simulink model "ModeloCodesys"  (R2020b)
settings: Solver=FixedStepAuto  StartTime=0.0  StopTime=inf  FixedStep=1e-2  MaxStep=1e-4  RelTol=1e-3
model workspace (MAT data in the model file):
  sensor_carga : Simulink.Parameter (value not decoded)
values from neighbouring files (symbols this model uses):
  bcx = 1000e3    (= 1000000)    [Datos_simulacion.m]
  bcy = 500e3    (= 500000)    [Datos_simulacion.m]
  beq_tc = (bv_c+beq_cel)/Rw^2    (= 27000)    [Datos_simulacion.m]
  beq_ti = (b_h+beq_iel)/Rd^2    (= 28800)    [Datos_simulacion.m]
  bw = 30e3    (= 30000)    [Datos_simulacion.m]
  g = 9.80665    [Datos_simulacion.m]
  i_c = 15    [Datos_simulacion.m]
  i_i = 30    [Datos_simulacion.m]
  Kcd = Meq_c*polo_c*n    (= 472500)    [Datos_simulacion.m]
  Kci = Kcp*polo_c/n    (= 1938936.66179)    [Datos_simulacion.m]
  Kcp = Kcd*polo_c    (= 1513396.48861)    [Datos_simulacion.m]
  Kcy = 1.3e9    (= 1300000000)    [Datos_simulacion.m]
  Kid = Kcp*polo_i/n    (= 1815537.84919)    [Datos_simulacion.m]
  Kii = Meq_i*polo_i*n    (= 360000)    [Datos_simulacion.m]
  Kip = Kcd*polo_i    (= 1417080.12441)    [Datos_simulacion.m]
  Kw = 1800e3    (= 1800000)    [Datos_simulacion.m]
  Meq_c = m_c+Jeq_c/Rw^2    (= 59008)    [Datos_simulacion.m]
  Meq_i = m_h+Jeq_i/Rd^2    (= 48014.2222222)    [Datos_simulacion.m]
  Rd = 0.75    [Datos_simulacion.m]
  Rw = 0.5    [Datos_simulacion.m]
  Tau = 1e-3    (= 0.001)    [Datos_simulacion.m]
libraries: simulink x2, fuzblock x1, pid_lib x1, dspswit3 x1
(part 2 of 2)

== matlab function ModeloCodesys/Algoritmos de busqueda de camino y interpolacion/Interpolador ==
  data: wayPoints input size=2,100; q output size=[2,1000000]; velMaxX input; velMaxY input
function q  = Interp(wayPoints,velMaxX,velMaxY)
coder.extrinsic('plot')
pendiente_ant=0;
cont_p=1;
wayPoints=wayPoints([2,1],:);
wayPoints=flip(wayPoints,2);
wayPoints(2,:)=(wayPoints(2,:)-65)*-1;
for i=1:length(wayPoints)-1
    pendiente=(wayPoints(2,i)-wayPoints(2,i+1))/(wayPoints(1,i)-wayPoints(1,i+1));
    if pendiente_ant~=pendiente
        cont_p=cont_p+1;
    end
    pendiente_ant=pendiente;
end
wayPoints1=zeros(2,cont_p);
cont_p2=0;
for i=1:length(wayPoints(1,:))-1
    pendiente=(wayPoints(2,i)-wayPoints(2,i+1))/(wayPoints(1,i)-wayPoints(1,i+1));
    if pendiente_ant~=pendiente
    cont_p2=cont_p2+1;
    wayPoints1(:,cont_p2)=wayPoints(:,i);
    end
    pendiente_ant=pendiente;
end
wayPoints1(:,end)=wayPoints(:,end);
wayPoints1(:,1)=wayPoints(:,1);
figure(10)
plot(wayPoints1(1,:),wayPoints1(2,:))   
vx_max=velMaxX;
vy_max=velMaxY;
timePoints1=zeros(1,length(wayPoints1));
tiempo_ant=0;
for i=1:length(wayPoints1(1,:))-1
    restaX=abs(wayPoints1(1,i+1)-wayPoints1(1,i));
    restaY=abs(wayPoints1(2,i+1)-wayPoints1(2,i));
    timex=restaX/(vx_max/2.5);
    timey=restaY/(vy_max/2.5);
    if timex>timey
    timePoints1(i+1)=restaX/(vx_max/4)+tiempo_ant;
    elseif timex<timey
    timePoints1(i+1)=restaY/(vy_max/4)+tiempo_ant;
    else
     timePoints1(i+1)=restaX/(vx_max/4)+tiempo_ant;    
    end
    tiempo_ant=timePoints1(i+1);
end
tSamples1=0:1e-2:timePoints1(end);
q = zeros(2,length(tSamples1));%'VelocityBoundaryCondition',vel_max);
qx=interp1(timePoints1,wayPoints1(1,:),tSamples1,'pchip');
qy=interp1(timePoints1,wayPoints1(2,:),tSamples1,'pchip');
q(1,:)=qx;
q(2,:)=qy;
figure(15)
plot(qx,qy)  

end
